simulink model "ev_charging_stations"  (Simulink 8.1)
settings: Solver=ode3  StartTime=0  StopTime=14400  FixedStep=1  RelTol=1e-3
undefined symbols (not defined in the file or in its folder): D1, Delta, Ts
libraries: CampusEnergyModeling x4, powerlib x4, powerlib_meascontrol x1
settings Model: Creator=sfrank1  LastModifiedBy=sfrank1
settings DataIOCC: SignalLoggingSaveFormat=Dataset
settings OptimizationCC: ExpressionDepthLimit=128
settings DebuggingCC: FcnCallInpInsideContextMsg=EnableAllAsError
settings GRTTargetCC: CombineOutputUpdateFcns=on  GRTInterface=off

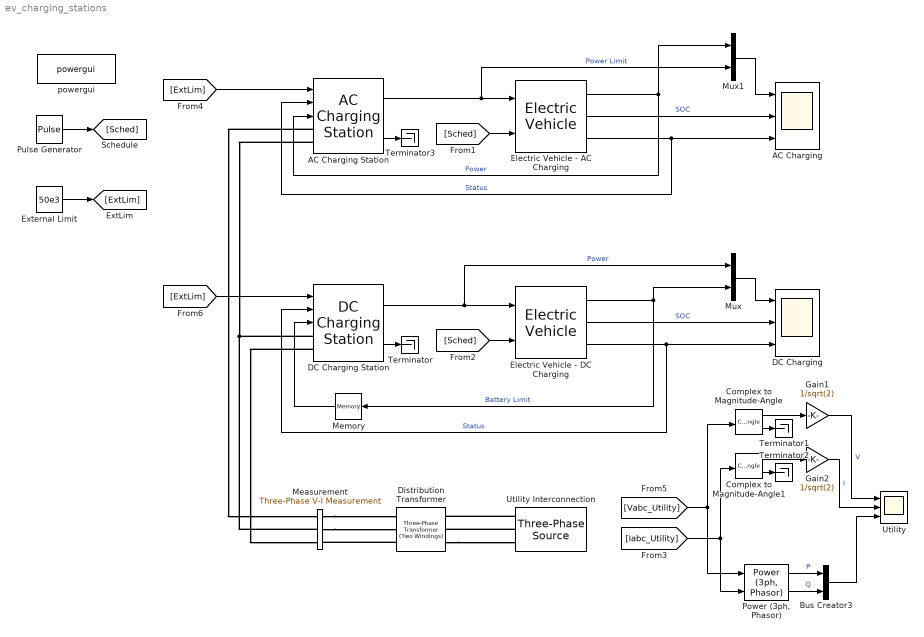
== system ev_charging_stations ==
  AC Charging : Scope  NumInputPorts=3
      settings: ShowLegends=on  TimeRange=15000  YMin=0~0~-1  YMax=6000~1~0
  AC Charging Station : CampusEnergyModeling/Electric Vehicles/AC Charging Station  prated=6000  vrated=240  pstandby=10  eff=0.99  pf=0.99  freq=60
  Bus Creator3 : BusCreator  Inputs=2
  Complex to Magnitude-Angle : ComplexToMagnitudeAngle
  Complex to Magnitude-Angle1 : ComplexToMagnitudeAngle
  DC Charging : Scope  NumInputPorts=3
      settings: ShowLegends=on  TimeRange=15000  YMin=0~0~-1  YMax=1000~1~0
  DC Charging Station : CampusEnergyModeling/Electric Vehicles/DC Charging Station  prated=24000  vrated=240  pstandby=100  eff=0.97  pf=0.99  freq=60
  Distribution Transformer : powerlib/Elements/Three-Phase Transformer (Two Windings)  Winding1Connection=Delta (D1)  UNITS=pu  NominalPower=[10e3 , 60]  Winding1=[13.2e3 , 0.02/2 , 0.05/(120*pi)/2]  Winding2Connection=Yg  Winding2=[208 , 0.02/2 , 0.05/(120*pi)/2]  SetSaturation=off  Rm=500  Lm=200  Saturation=[ 0,0 ; 0.0024,1.2 ; 1.0,1.52 ]  Hysteresis=off  DataFile='hysteresis'  SetInitialFlux=off  InitialFluxes=[ 0.8 , -0.8 , 0.7 ]  Measurements=None  MoreParameters=off  BreakLoop=off  DataType=off  TransfoNumber=1
  Electric Vehicle - AC Charging : CampusEnergyModeling/Electric Vehicles/Electric Vehicle  ctype=AC  rating=1000  chargerEff=0.98  profile=off  profileSOC=[0.00 0.10 0.20 0.80 0.99 1.00]  profileRate=[0.10 0.20 1.00 1.00 0.01 0.00]  capacity=1000  initSOC=0  battEff=0.98
  Electric Vehicle - DC Charging : CampusEnergyModeling/Electric Vehicles/Electric Vehicle  ctype=DC  rating=6240  chargerEff=0.96  profile=off  profileSOC=[0.00 0.10 0.20 0.80 0.99 1.00]  profileRate=[0.10 0.20 1.00 1.00 0.01 0.00]  capacity=1000  initSOC=0  battEff=0.98
  External Limit : Constant  Value=50e3
  Gain1 : Gain  Gain=1/sqrt(2)
  Gain2 : Gain  Gain=1/sqrt(2)
  Measurement : powerlib/Measurements/Three-Phase V-I Measurement  VoltageMeasurement=phase-to-ground  SetLabelV=on  LabelV=Vabc_Utility  Vpu=off  VpuLL=off  CurrentMeasurement=yes  SetLabelI=on  LabelI=Iabc_Utility  Ipu=off  Pbase=10e3  Vbase=208  OutputType=Complex  PhasorSimulation=on  PSBequivalent=0
  Memory : Memory
  Mux : Mux  Inputs=2
  Mux1 : Mux  Inputs=2
  "Power (3ph, Phasor)" : powerlib_meascontrol/Measurements/Power (3ph, Phasor)
  Pulse Generator : DiscretePulseGenerator  PulseType=Time based  Period=9000  PulseWidth=90  PhaseDelay=1800
  Terminator{,1..3} (4 alike) : Terminator
  Utility : Scope  NumInputPorts=3
      settings: ShowLegends=on  TimeRange=15000  YMin=112~0~0  YMax=121~20.51886792452825~4988.262910798119  SaveName=ScopeData2
  Utility Interconnection : powerlib/Electrical Sources/Three-Phase Source  Voltage=13.2e3  PhaseAngle=0  Frequency=60  InternalConnection=Yg  SpecifyImpedance=on  Resistance=0.8929  Inductance=16.58e-3  ShortCircuitLevel=1e6  BaseVoltage=13.2e3  XRratio=8  BusType=swing  Pref=0  Qref=0  Qmin=-inf  Qmax=inf
  powergui : powerlib/powergui  Priority=2  SimulationMode=Phasor  SolverType=Tustin  SampleTime=Ts  frequency=60  SPID=off  DisableSnubberDevices=off  DisableRonSwitches=off  DisableVfSwitches=off  SwTol=0  Interpol=off  DisplayEquations=off  frequencyindice=60  Pbase=100e6  ErrMax=1e-4  Iterations=50  UnitsV=kV  UnitsW=kW  FunctionMessages=off  echomessages=off  HookPort=off  EnableUseOfTLC=off  x0status=blocks  RestoreLinks=warning  ResistiveCurrentMeasurement=off  Frange=[0:2:500]  Ylog=off  Xlog=on  ShowGrid=off  save=off  variable=ZData  structure=Sig1  ZoomFFT=on  StartTime=0.26  cycles=2  DisplayStyle=1  fundamental=60  FreqAxis=off  MaxFrequency=5000  frequencyindicesteady=1  RmsSteady=1  display=off  Ts=0  methode=off
  wires:
  Electric Vehicle - DC Charging/1 -> Memory/1, Mux/2  "Battery Limit"
  DC Charging Station/1 -> Mux/1, Electric Vehicle - DC Charging/1  "Power"
  Mux/1 -> DC Charging/1
  Electric Vehicle - DC Charging/2 -> DC Charging/2  "SOC"
  Electric Vehicle - DC Charging/3 -> DC Charging Station/2, DC Charging/3  "Status"
  Mux1/1 -> AC Charging/1
  Electric Vehicle - AC Charging/2 -> AC Charging/2  "SOC"
  Electric Vehicle - AC Charging/3 -> AC Charging Station/2, AC Charging/3  "Status"
  Electric Vehicle - AC Charging/1 -> AC Charging Station/3, Mux1/1  "Power"
  [Sched] -> Electric Vehicle - AC Charging/2
  Pulse Generator/1 -> [Sched]
  [Sched] -> Electric Vehicle - DC Charging/2
  [Vabc_Utility] -> Complex to Magnitude-Angle/1, "Power (3ph, Phasor)"/1
  [Iabc_Utility] -> Complex to Magnitude-Angle1/1, "Power (3ph, Phasor)"/2
  AC Charging Station/1 -> Mux1/2, Electric Vehicle - AC Charging/1  "Power Limit"
  External Limit/1 -> [ExtLim]
  [ExtLim] -> AC Charging Station/1
  [ExtLim] -> DC Charging Station/1
  DC Charging Station/2 -> Terminator/1
  Memory/1 -> DC Charging Station/3
  "Power (3ph, Phasor)"/2 -> Bus Creator3/2  "Q"
  "Power (3ph, Phasor)"/1 -> Bus Creator3/1  "P"
  Bus Creator3/1 -> Utility/3
  Gain1/1 -> Utility/1  "V"
  Gain2/1 -> Utility/2  "I"
  Complex to Magnitude-Angle/2 -> Terminator1/1
  Complex to Magnitude-Angle/1 -> Gain1/1
  Complex to Magnitude-Angle1/2 -> Terminator2/1
  Complex to Magnitude-Angle1/1 -> Gain2/1
  AC Charging Station/2 -> Terminator3/1
  connections:
  Utility Interconnection/RConn2 -- Distribution Transformer/LConn2
  Utility Interconnection/RConn1 -- Distribution Transformer/LConn1
  Distribution Transformer/LConn3 -- Utility Interconnection/RConn3
  Measurement/RConn2 -- DC Charging Station/LConn1 -- AC Charging Station/LConn2
  Distribution Transformer/RConn3 -- Measurement/LConn3
  Measurement/LConn2 -- Distribution Transformer/RConn2
  Measurement/LConn1 -- Distribution Transformer/RConn1
  AC Charging Station/LConn1 -- Measurement/RConn1
  DC Charging Station/LConn2 -- Measurement/RConn3
